simulink model "SAR_Quad_SITL_3D_v3"  (R2025b)
settings: Solver=ode4  StartTime=0.0  StopTime=inf  FixedStep=1/60  RelTol=1e-3
libraries: dspnetwork x5, sim3dlib x1, uavsim3dlib x1
(part 1 of 2)
settings Model: Creator=User  LastModifiedBy=User

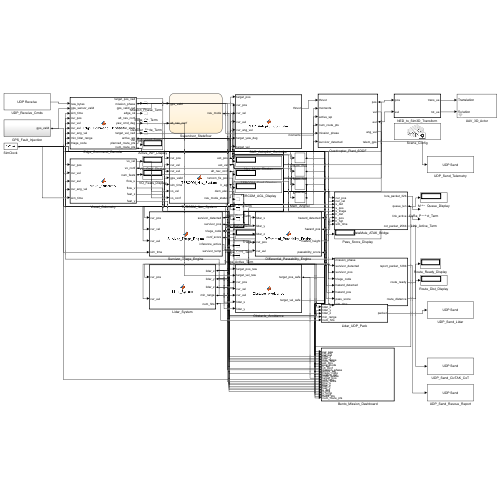
[thumbnail: Simulink's stored preview of the top-level diagram]
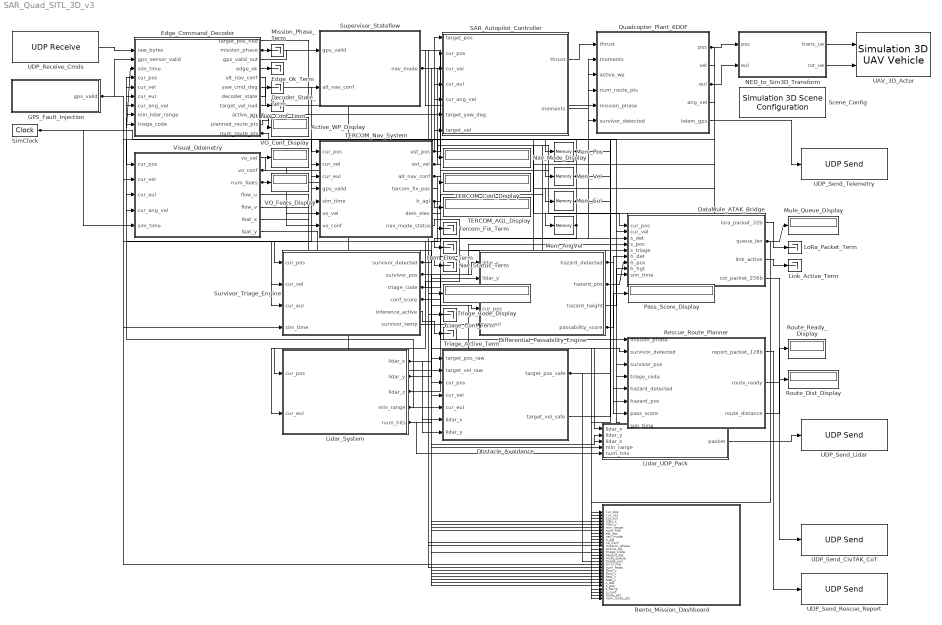
== system SAR_Quad_SITL_3D_v3 ==
  Active_WP_Display : Display
  Alt_Nav_Conf_Term : Terminator
  Bento_Mission_Dashboard : MATLAB Function  TreatAsAtomicUnit=on
  DataMule_ATAK_Bridge : MATLAB Function  TreatAsAtomicUnit=on
  Decoder_State_Term : Terminator
  Dem_Elev_Term : Terminator
  Differential_Passability_Engine : MATLAB Function  TreatAsAtomicUnit=on
  Edge_Command_Decoder : MATLAB Function  TreatAsAtomicUnit=on
  Edge_Ok_Term : Terminator
  GPS_Fault_Injection : Subsystem
  Lidar_System : MATLAB Function  TreatAsAtomicUnit=on
  Lidar_UDP_Pack : MATLAB Function  TreatAsAtomicUnit=on
  Link_Active_Term : Terminator
  LoRa_Packet_Term : Terminator
  Mem_AngVel : Memory  InitialCondition=[0; 0; 0]
  Mem_Eul : Memory  InitialCondition=[0; 0; 0]
  Mem_Pos : Memory  InitialCondition=[0; 0; 0]
  Mem_Vel : Memory  InitialCondition=[0; 0; 0]
  Mission_Phase_Term : Terminator
  Mule_Queue_Display : Display
  NED_to_Sim3D_Transform : MATLAB Function  TreatAsAtomicUnit=on
  Nav_Mode_Display : Display
  Nav_Status_Term : Terminator
  Obstacle_Avoidance : MATLAB Function  TreatAsAtomicUnit=on
  Pass_Score_Display : Display
  Quadcopter_Plant_6DOF : MATLAB Function  TreatAsAtomicUnit=on
  Rescue_Route_Planner : MATLAB Function  TreatAsAtomicUnit=on
  Route_Dist_Display : Display
  Route_Ready_Display : Display
  SAR_Autopilot_Controller : MATLAB Function  TreatAsAtomicUnit=on
  Scene_Config : sim3dlib/Simulation 3D Scene Configuration  Priority=0  ProjectFormat=Default Scenes  SceneDesc=US city block  ProjectName=D:\MLAB\toolbox\shared\sim3d_projects\automotive_project_windows\UE\WindowsNoEditor\VehicleSimulation.exe  ScenePath=/Game/Maps/USCityBlock  EnableOpenDRIVE=off  vehTagList={'Custom';'Scene Origin'}  vehTag=Scene Origin  AttachedCameraRelativeTranslation=[0 0 0]  FreeCameraDefaultInitialTranslation=[-6, 0, 2]  AttachedCameraRelativeRotation=[0 0 0]  FreeCameraDefaultInitialRotation=[0, -15, 0]  ViewpointName=Custom  FreeCameraInitialTranslation=[0, 0, 0]  ViewpointTranslation=[0, 0, 0]  FreeCameraInitialRotation=[0, 0, 0]  ViewpointRotation=[0, 0, 0]  OpVisEn=off  Ts=1/60  EnableWindow=on  EnableRemoteAccess=off  EnableWeather=off  SunAzimuth=90  SunAltitude=40.0  EnableGeospatialSun=off  Latitude=0  Longitude=0  Date=2023-01-01  Time=10:30:00  GeoTimeZone=-5.0  SunDaylightSaving=off  wind=1  clouds=10  EnableVolumetricClouds=off  CloudCoverage=0  CloudAltitude=6  fog=0  rain=0  RaindropsEffect=off  SnowDensity=0  EnableGeospatial=off  TilesetSource=Earth terrain  UseTrueOrigin=off  OriginHeight=200  OriginLatitude=40.744652  OriginLongitude=-73.988864  MapStyle=Aerial  AdditionalAssetIDs=[]  UseAdvancedSunSky=off  SolarTime=11  TimeZone=-5  Day=21  Month=9  Year=2022  UseDaylightSavingTime=on  DSTStartDay=10  DSTStartMonth=3  DSTEndDay=3  DSTEndMonth=11  DSTSwitchHour=2  sensorTag=MainCamera1  sensorId=1  sensorName=MainCamera1  mountLoc=Origin  offsetFlag=off  tmountOffset=[0, 0, 0]  rmountOffset=[0, 0, 0]  HorizontalResolution=1280  VerticalResolution=720  HorizontalFOV=60  mountPoint=[0 0 0]  mountOrientation=[0 0 0]  aMode=4  ID=1  GeoTrigger=Inactive  ViewNameList={'Custom'}  ViewTranslationList={'[0 0 0]'}  ViewRotationList={'[0 0 0]'}
      settings: LibrarySourceBlock=uavsim3dlib/Simulation 3D Scene Configuration
  SimClock : DigitalClock  SampleTime=1/60
  Supervisor_Stateflow : Stateflow chart  TreatAsAtomicUnit=on
  Survivor_Triage_Engine : MATLAB Function  TreatAsAtomicUnit=on
  TERCOM_AGL_Display : Display
  TERCOM_Conf_Display : Display
  TERCOM_Nav_System : MATLAB Function  TreatAsAtomicUnit=on
  Tercom_Fix_Term : Terminator
  Triage_Active_Term : Terminator
  Triage_Code_Display : Display
  Triage_Conf_Term : Terminator
  UAV_3D_Actor : uavsim3dlib/Simulation 3D UAV Vehicle  Priority=-1  Mesh=Quadrotor  MeshPath=/MathWorksUAVContent/UAVs/HexaRotorUAV/HexaRotor.HexaRotor  Color=Black  ActorName=SimulinkVehicle1  UseGlobalFrame=off  InitialTranslation=[0 0 0]  InitialRotation=[0 0 0]  InitialTranslationGlobal=[0 0 0]  InitialGeoOrigin=[0 0 0]  InitialRotationGlobal=[0 0 0]  SampleTime=-1  ActorType=SimulinkVehicle  ID=1  aMode=4  ActorTag=SimulinkVehicle1
  UDP_Receive_Cmds : dspnetwork/UDP Receive  localURL='0.0.0.0'  localPort=5001  remoteURL='0.0.0.0'  remotePort=-1  recvBufferSize=8192  dims=255  signalDatatype=uint8  isComplex=off  isVarSize=on  showBlockingTime=off  blockingTime=0  sampletime=1/60  blockPlatform=[]
  UDP_Send_CivTAK_CoT : dspnetwork/UDP Send  remoteURL='127.0.0.1'  remotePort=4242  localURL='0.0.0.0'  localPortSource=Automatically determine  localPort=2048  sendBufferSize=8192  sampletime=-1  blockPlatform=[]  separateLengthPort=0
  UDP_Send_Lidar : dspnetwork/UDP Send  remoteURL='127.0.0.1'  remotePort=5003  localURL='0.0.0.0'  localPortSource=Automatically determine  localPort=2048  sendBufferSize=8192  sampletime=-1  blockPlatform=[]  separateLengthPort=0
  UDP_Send_Rescue_Report : dspnetwork/UDP Send  remoteURL='127.0.0.1'  remotePort=4243  localURL='0.0.0.0'  localPortSource=Automatically determine  localPort=2048  sendBufferSize=8192  sampletime=-1  blockPlatform=[]  separateLengthPort=0
  UDP_Send_Telemetry : dspnetwork/UDP Send  remoteURL='127.0.0.1'  remotePort=5002  localURL='0.0.0.0'  localPortSource=Automatically determine  localPort=2048  sendBufferSize=8192  sampletime=-1  blockPlatform=[]  separateLengthPort=0
  VO_Conf_Display : Display
  VO_Feats_Display : Display
  Visual_Odometry : MATLAB Function  TreatAsAtomicUnit=on
  wires:
  UDP_Receive_Cmds/1 -> Edge_Command_Decoder/1(raw_bytes)
  GPS_Fault_Injection/1(gps_valid) -> Edge_Command_Decoder/2(gps_sensor_valid), TERCOM_Nav_System/4(gps_valid)
  SimClock/1 -> Edge_Command_Decoder/3(sim_time), Visual_Odometry/5(sim_time), TERCOM_Nav_System/5(sim_time), Survivor_Triage_Engine/4(sim_time), DataMule_ATAK_Bridge/9(sim_time), Rescue_Route_Planner/8(sim_time), Bento_Mission_Dashboard/18(sim_time)
  TERCOM_Nav_System/1(est_pos) -> Edge_Command_Decoder/4(cur_pos), Survivor_Triage_Engine/1(cur_pos), Differential_Passability_Engine/4(cur_pos), DataMule_ATAK_Bridge/1(cur_pos), Obstacle_Avoidance/3(cur_pos), SAR_Autopilot_Controller/2(cur_pos), Bento_Mission_Dashboard/8(est_pos)
  TERCOM_Nav_System/2(est_vel) -> Edge_Command_Decoder/5(cur_vel), Survivor_Triage_Engine/2(cur_vel), DataMule_ATAK_Bridge/2(cur_vel), Obstacle_Avoidance/4(cur_vel), SAR_Autopilot_Controller/3(cur_vel)
  Mem_Eul/1 -> Edge_Command_Decoder/6(cur_eul), Visual_Odometry/3(cur_eul), TERCOM_Nav_System/3(cur_eul), Survivor_Triage_Engine/3(cur_eul), Differential_Passability_Engine/5(cur_eul), Obstacle_Avoidance/5(cur_eul), SAR_Autopilot_Controller/4(cur_eul), Lidar_System/2(cur_eul), Bento_Mission_Dashboard/3(cur_eul)
  Mem_AngVel/1 -> Edge_Command_Decoder/7(cur_ang_vel), Visual_Odometry/4(cur_ang_vel), SAR_Autopilot_Controller/5(cur_ang_vel)
  Lidar_System/4(min_range) -> Edge_Command_Decoder/8(min_lidar_range), Lidar_UDP_Pack/4(min_range), Bento_Mission_Dashboard/6(min_range)
  Survivor_Triage_Engine/3(triage_code) -> Edge_Command_Decoder/9(triage_code), Triage_Code_Display/1, DataMule_ATAK_Bridge/5(s_triage), Rescue_Route_Planner/4(triage_code), Bento_Mission_Dashboard/14(triage_code)
  Edge_Command_Decoder/2(mission_phase) -> Mission_Phase_Term/1, Rescue_Route_Planner/1(mission_phase), Quadcopter_Plant_6DOF/5(mission_phase), Bento_Mission_Dashboard/12(mission_phase)
  Edge_Command_Decoder/3(gps_valid_out) -> Supervisor_Stateflow/1(gps_valid)
  Edge_Command_Decoder/4(edge_ok) -> Edge_Ok_Term/1
  Edge_Command_Decoder/5(alt_nav_conf) -> Alt_Nav_Conf_Term/1
  Edge_Command_Decoder/7(decoder_state) -> Decoder_State_Term/1
  Edge_Command_Decoder/9(active_wp) -> Active_WP_Display/1, Quadcopter_Plant_6DOF/3(active_wp), Bento_Mission_Dashboard/13(active_wp)
  Supervisor_Stateflow/1(nav_mode) -> Nav_Mode_Display/1, Bento_Mission_Dashboard/9(nav_mode)
  TERCOM_Nav_System/3(alt_nav_conf) -> Supervisor_Stateflow/2(alt_nav_conf), TERCOM_Conf_Display/1
  Mem_Pos/1 -> Visual_Odometry/1(cur_pos), TERCOM_Nav_System/1(cur_pos), Lidar_System/1(cur_pos), Bento_Mission_Dashboard/1(cur_pos)
  Mem_Vel/1 -> Visual_Odometry/2(cur_vel), TERCOM_Nav_System/2(cur_vel), Bento_Mission_Dashboard/2(cur_vel)
  Visual_Odometry/2(vo_conf) -> VO_Conf_Display/1, TERCOM_Nav_System/7(vo_conf), Bento_Mission_Dashboard/11(vo_conf)
  Visual_Odometry/3(num_feats) -> VO_Feats_Display/1, Bento_Mission_Dashboard/19(num_feats)
  Visual_Odometry/1(vo_vel) -> TERCOM_Nav_System/6(vo_vel)
  TERCOM_Nav_System/4(tercom_fix_pos) -> Tercom_Fix_Term/1
  TERCOM_Nav_System/5(h_agl) -> TERCOM_AGL_Display/1, Bento_Mission_Dashboard/10(h_agl)
  TERCOM_Nav_System/6(dem_elev) -> Dem_Elev_Term/1
  TERCOM_Nav_System/7(nav_mode_status) -> Nav_Status_Term/1
  Survivor_Triage_Engine/4(conf_score) -> Triage_Conf_Term/1, Bento_Mission_Dashboard/27(s_conf)
  Survivor_Triage_Engine/5(inference_active) -> Triage_Active_Term/1
  Lidar_System/1(lidar_x) -> Differential_Passability_Engine/1(lidar_x), Obstacle_Avoidance/6(lidar_x), Lidar_UDP_Pack/1(lidar_x), Bento_Mission_Dashboard/4(lidar_x)
  Lidar_System/2(lidar_y) -> Differential_Passability_Engine/2(lidar_y), Obstacle_Avoidance/7(lidar_y), Lidar_UDP_Pack/2(lidar_y), Bento_Mission_Dashboard/5(lidar_y)
  Lidar_System/3(lidar_z) -> Differential_Passability_Engine/3(lidar_z), Lidar_UDP_Pack/3(lidar_z)
  Differential_Passability_Engine/4(passability_score) -> Pass_Score_Display/1, Rescue_Route_Planner/7(pass_score)
  Survivor_Triage_Engine/1(survivor_detected) -> DataMule_ATAK_Bridge/3(s_det), Rescue_Route_Planner/2(survivor_detected), Quadcopter_Plant_6DOF/6(survivor_detected), Bento_Mission_Dashboard/24(s_det)
  Survivor_Triage_Engine/2(survivor_pos) -> DataMule_ATAK_Bridge/4(s_pos), Rescue_Route_Planner/3(survivor_pos), Bento_Mission_Dashboard/25(s_pos)
  Differential_Passability_Engine/1(hazard_detected) -> DataMule_ATAK_Bridge/6(h_det), Rescue_Route_Planner/5(hazard_detected), Bento_Mission_Dashboard/15(hazard_det)
  Differential_Passability_Engine/2(hazard_pos) -> DataMule_ATAK_Bridge/7(h_pos), Rescue_Route_Planner/6(hazard_pos)
  Differential_Passability_Engine/3(hazard_height) -> DataMule_ATAK_Bridge/8(h_hgt)
  DataMule_ATAK_Bridge/1(lora_packet_32b) -> LoRa_Packet_Term/1
  DataMule_ATAK_Bridge/2(queue_len) -> Mule_Queue_Display/1, Bento_Mission_Dashboard/16(mule_queue)
  DataMule_ATAK_Bridge/3(link_active) -> Link_Active_Term/1
  DataMule_ATAK_Bridge/4(cot_packet_256b) -> UDP_Send_CivTAK_CoT/1
  Rescue_Route_Planner/1(report_packet_128b) -> UDP_Send_Rescue_Report/1
  Rescue_Route_Planner/2(route_ready) -> Route_Ready_Display/1
  Rescue_Route_Planner/3(route_distance) -> Route_Dist_Display/1
  Edge_Command_Decoder/1(target_pos_ned) -> Obstacle_Avoidance/1(target_pos_raw)
  Edge_Command_Decoder/8(target_vel_ned) -> Obstacle_Avoidance/2(target_vel_raw)
  Obstacle_Avoidance/1(target_pos_safe) -> SAR_Autopilot_Controller/1(target_pos), Bento_Mission_Dashboard/17(target_pos)
  Edge_Command_Decoder/6(yaw_cmd_deg) -> SAR_Autopilot_Controller/6(target_yaw_deg)
  Obstacle_Avoidance/2(target_vel_safe) -> SAR_Autopilot_Controller/7(target_vel)
  SAR_Autopilot_Controller/1(thrust) -> Quadcopter_Plant_6DOF/1(thrust)
  SAR_Autopilot_Controller/2(moments) -> Quadcopter_Plant_6DOF/2(moments)
  Edge_Command_Decoder/11(num_route_pts) -> Quadcopter_Plant_6DOF/4(num_route_pts), Bento_Mission_Dashboard/29(num_route_pts)
  Quadcopter_Plant_6DOF/1(pos) -> Mem_Pos/1, NED_to_Sim3D_Transform/1(pos)
  Quadcopter_Plant_6DOF/2(vel) -> Mem_Vel/1
  Quadcopter_Plant_6DOF/3(eul) -> Mem_Eul/1, NED_to_Sim3D_Transform/2(eul)
  Quadcopter_Plant_6DOF/4(ang_vel) -> Mem_AngVel/1
  Lidar_System/5(num_hits) -> Lidar_UDP_Pack/5(num_hits), Bento_Mission_Dashboard/7(num_hits)
  Lidar_UDP_Pack/1(packet) -> UDP_Send_Lidar/1
  NED_to_Sim3D_Transform/1(trans_ue) -> UAV_3D_Actor/1
  NED_to_Sim3D_Transform/2(rot_ue) -> UAV_3D_Actor/2
  Quadcopter_Plant_6DOF/5(telem_gps) -> UDP_Send_Telemetry/1
  Visual_Odometry/4(flow_u) -> Bento_Mission_Dashboard/20(flow_u)
  Visual_Odometry/5(flow_v) -> Bento_Mission_Dashboard/21(flow_v)
  Visual_Odometry/6(feat_x) -> Bento_Mission_Dashboard/22(feat_x)
  Visual_Odometry/7(feat_y) -> Bento_Mission_Dashboard/23(feat_y)
  Survivor_Triage_Engine/6(survivor_temp) -> Bento_Mission_Dashboard/26(s_temp)
  Edge_Command_Decoder/10(planned_route_pts) -> Bento_Mission_Dashboard/28(route_pts)

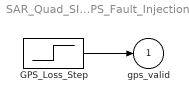
== system SAR_Quad_SITL_3D_v3/GPS_Fault_Injection ==
  GPS_Loss_Step : Step  Time=160  Before=1  After=0  SampleTime=1/60
  gps_valid : Outport
  wires:
  ? -> ?
  GPS_Loss_Step/1 -> gps_valid/1

== matlab function SAR_Quad_SITL_3D_v3/Survivor_Triage_Engine ==
  data: cur_pos input; survivor_detected output size=1; cur_vel input; cur_eul input; sim_time input; survivor_pos output size=3; triage_code output size=1; conf_score output size=1; inference_active output size=1; survivor_temp output size=1
function [survivor_detected, survivor_pos, triage_code, conf_score, inference_active, survivor_temp] = Survivor_Triage_Engine(cur_pos, cur_vel, cur_eul, sim_time)
survivor_detected = 0.0;
survivor_pos = [0.0; 0.0; 0.0];
triage_code = 0.0; conf_score = 0.0; inference_active = 0.0;
AMBIENT_TEMP = 22.0;
survivor_temp = AMBIENT_TEMP;
persistent survivors
if isempty(survivors)
    survivors = [
        145.0,  50.0, 0.0, 38.2, 1.0;   % Park Sector Target Actor (RED IMMEDIATE)
         22.0,   5.5, 0.0, 37.4, 1.0;   % Sector 1: Immediate Critical (RED)
        120.0, -35.0, 0.0, 36.8, 2.0;   % Sector 2: Delayed Triage (YELLOW)
         50.0,  18.0, 0.0, 36.9, 3.0    % Sector 3: Minor Injury (GREEN)
    ];
end
h_agl = max(1.0, -cur_pos(3));
r_footprint = max(4.5, h_agl * tan(35.0 * pi / 180));
v_ground = norm(cur_vel(1:2));

for i = 1:size(survivors, 1)
    d_xy = norm(survivors(i, 1:2) - cur_pos(1:2)');
    if d_xy <= r_footprint && h_agl >= 1.5
        inference_active = 1.0;
        survivor_detected = 1.0;
        survivor_pos = survivors(i, 1:3)';
        triage_code = survivors(i, 5);
        survivor_temp = survivors(i, 4);
        conf_score = max(0.60, 0.98 - 0.03 * (d_xy / r_footprint) - 0.01 * v_ground);
        break;
    end
end

== matlab function SAR_Quad_SITL_3D_v3/Differential_Passability_Engine ==
  data: lidar_x input; hazard_detected output size=1; lidar_y input; lidar_z input; cur_pos input; cur_eul input; hazard_pos output size=3; hazard_height output size=1; passability_score output size=1
function [hazard_detected, hazard_pos, hazard_height, passability_score] = Differential_Passability_Engine(lidar_x, lidar_y, lidar_z, cur_pos, cur_eul)
hazard_detected = 0.0;
hazard_pos = [0.0; 0.0; 0.0];
hazard_height = 0.0;
passability_score = 1.0;
yaw = cur_eul(3); c = cos(yaw); s = sin(yaw);
wx = cur_pos(1) + c .* lidar_x - s .* lidar_y;
wy = cur_pos(2) + s .* lidar_x + c .* lidar_y;
wz = -cur_pos(3) + lidar_z;
N = numel(lidar_x);
max_delta = 0.0; best_hx = 0.0; best_hy = 0.0;
for i = 1:min(N, 72)
    is_road = (abs(wy(i)) <= 7.5) || (abs(wx(i) - 120.0) <= 7.5) || (abs(wx(i) - 50.0) <= 4.0) || (abs(wx(i) + 20.0) <= 7.5);
    if is_road && wz(i) > 0.35 && wz(i) < 4.0
        if wz(i) > max_delta
            max_delta = wz(i); best_hx = wx(i); best_hy = wy(i);
        end
    end
end
if max_delta > 0.40
    hazard_detected = 1.0;
    hazard_pos = [best_hx; best_hy; max_delta];
    hazard_height = max_delta;
    passability_score = max(0.0, 1.0 - (max_delta / 3.0));
end

== matlab function SAR_Quad_SITL_3D_v3/DataMule_ATAK_Bridge ==
  data: cur_pos input; lora_packet_32b output size=32; cur_vel input; s_det input; s_pos input; s_triage input; h_det input; h_pos input; h_hgt input; sim_time input; queue_len output size=1; link_active output size=1; cot_packet_256b output size=256
function [lora_packet_32b, queue_len, link_active, cot_packet_256b] = DataMule_ATAK_Bridge(cur_pos, cur_vel, s_det, s_pos, s_triage, h_det, h_pos, h_hgt, sim_time)
lora_packet_32b = zeros(32, 1, 'uint8');
cot_packet_256b = zeros(256, 1, 'uint8');
link_active = 0.0;
persistent queue_count cot_count
if isempty(queue_count)
    queue_count = 0.0; cot_count = 0.0;
end
if norm(cur_pos(1:2)) < 40.0; link_active = 1.0; end
if s_det > 0.5 || h_det > 0.5; queue_count = min(64.0, queue_count + 0.05); end
if link_active > 0.5 && queue_count > 0.1
    queue_count = max(0.0, queue_count - 0.25);
    cot_count   = cot_count + 1.0;
end

lora_packet_32b(1) = uint8(170);
lora_packet_32b(2) = uint8(s_triage);
lora_packet_32b(3) = uint8(round(min(30.0, norm(cur_vel(1:2))) * 10));
lora_packet_32b(4) = uint8(round(min(50.0, -cur_pos(3))));
lora_packet_32b(5) = uint8(round(h_hgt * 10));
lora_packet_32b(6) = uint8(mod(round(sim_time), 255));
lora_packet_32b(7) = uint8(round(max(0.0, min(100.0, 98.0 - sim_time * 0.05))));

cot_msg = sprintf('<event version="2.0" uid="SAR-UAV-01" type="a-f-G-U-C" how="m-g" time="%.0f" start="%.0f" stale="%.0f"><point lat="26.9948" lon="88.2854" hae="%.1f" ce="1.5" le="1.0"/><detail><triage code="%.0f"/><contact callsign="RESCUE-BRAIN-01"/></detail></event>', sim_time, sim_time, sim_time + 30, -cur_pos(3), s_triage);
bytes = uint8(cot_msg);
n = min(numel(bytes), 256);
cot_packet_256b(1:n) = bytes(1:n);
queue_len = queue_count;

== matlab function SAR_Quad_SITL_3D_v3/Rescue_Route_Planner ==
  data: mission_phase input; report_packet_128b output size=128; survivor_detected input; survivor_pos input; triage_code input; hazard_detected input; hazard_pos input; pass_score input; sim_time input; route_ready output size=1; route_distance output size=1
function [report_packet_128b, route_ready, route_distance] = Rescue_Route_Planner(mission_phase, survivor_detected, survivor_pos, triage_code, hazard_detected, hazard_pos, pass_score, sim_time)
report_packet_128b = zeros(128, 1, 'uint8');
route_ready = 0.0; route_distance = 0.0;
MAX_WP = 6; route_pts = zeros(MAX_WP, 2); num_pts = 0.0;
if mission_phase >= 1.0 || survivor_detected > 0.5
    route_ready = 1.0;
    dest_north = 145.0; dest_east = 50.0;
    if survivor_detected > 0.5
        dest_north = survivor_pos(1); dest_east = survivor_pos(2);
    end
    p_base = [0.0, 0.0]; p_target = [dest_north, dest_east];
    detour_needed = false;
    if hazard_detected > 0.5
        if norm(hazard_pos(1:2) - [60.0; 0.0]) < 10.0; detour_needed = true; end
    end
    if detour_needed
        route_pts(1, :) = p_base; route_pts(2, :) = [20.0, -4.5]; route_pts(3, :) = [120.0, -4.5]; route_pts(4, :) = p_target;
        num_pts = 4.0; mode_flag = 2.0;
    else
        route_pts(1, :) = p_base; route_pts(2, :) = [dest_north, 0.0]; route_pts(3, :) = p_target;
        num_pts = 3.0; mode_flag = 1.0;
    end
    total_d = 0.0;
    for i = 1:(int32(num_pts) - 1)
        total_d = total_d + norm(route_pts(i+1, :) - route_pts(i, :));
    end
    route_distance = total_d;
    msg = sprintf('RPT:INGRESS|TGT:%.0f,%.0f|TRG:%.0f|DIST:%.1fm|DETOUR:%.0f|WP_CNT:%.0f|TIME:%.0f', dest_north, dest_east, triage_code, route_distance, mode_flag, num_pts, sim_time);
    b_str = uint8(msg); n_len = min(numel(b_str), 128);
    report_packet_128b(1:n_len) = b_str(1:n_len);
end

== matlab function SAR_Quad_SITL_3D_v3/SAR_Autopilot_Controller ==
  data: target_pos input; thrust output size=1; cur_pos input; cur_vel input; cur_eul input; cur_ang_vel input; target_yaw_deg input; target_vel input; moments output size=3
function [thrust, moments] = SAR_Autopilot_Controller(target_pos, cur_pos, cur_vel, cur_eul, cur_ang_vel, target_yaw_deg, target_vel)
thrust = 0.0; moments = [0.0; 0.0; 0.0];
persistent int_vel_err int_att_err int_z_err
persistent pitch_cmd_filt roll_cmd_filt
if isempty(int_vel_err)
    int_vel_err = [0.0; 0.0]; int_att_err = [0.0; 0.0; 0.0]; int_z_err = 0.0;
    pitch_cmd_filt = 0.0; roll_cmd_filt = 0.0;
end

if cur_pos(3) >= -0.05 && target_pos(3) >= -0.05
    thrust = 0.0;
    moments = [0.0; 0.0; 0.0];
    int_vel_err = [0.0; 0.0]; int_att_err = [0.0; 0.0; 0.0]; int_z_err = 0.0;
    pitch_cmd_filt = 0.0; roll_cmd_filt = 0.0;
    return;
end

dt = 1/60; m = 1.8; g = 9.81;

% REALISTIC TACTICAL TILT LIMIT (20 DEGREES)
kp_p = 1.90; kp_v = 3.40; ki_v = 0.14;
e_pos_xy = target_pos(1:2) - cur_pos(1:2);
e_vel_xy = target_vel(1:2) - cur_vel(1:2);
int_vel_err = max(min(int_vel_err + (e_vel_xy * dt), 0.8), -0.8);

acc_world = kp_p * e_pos_xy + kp_v * e_vel_xy + ki_v * int_vel_err;
yaw_now = cur_eul(3);
acc_body_x =  acc_world(1) * cos(yaw_now) + acc_world(2) * sin(yaw_now);
acc_body_y = -acc_world(1) * sin(yaw_now) + acc_world(2) * cos(yaw_now);

MAX_TILT = 20.0 * pi / 180.0; % Hard mechanical bank ceiling
pitch_cmd_raw = max(min(-acc_body_x / g, MAX_TILT), -MAX_TILT);
roll_cmd_raw  = max(min( acc_body_y / g, MAX_TILT), -MAX_TILT);

% TILT FILTER (Smooth 10 Hz roll/pitch response)
alpha_tilt = 0.14;
pitch_cmd_filt = (1.0 - alpha_tilt) * pitch_cmd_filt + alpha_tilt * pitch_cmd_raw;
roll_cmd_filt  = (1.0 - alpha_tilt) * roll_cmd_filt  + alpha_tilt * roll_cmd_raw;

kp_z = 7.50; ki_z = 0.60; kd_z = 3.80;
e_pos_z = target_pos(3) - cur_pos(3);
e_vel_z = target_vel(3) - cur_vel(3);
int_z_err = max(min(int_z_err + (e_pos_z * dt), 1.2), -1.2);
az_pid = kp_z * e_pos_z + kd_z * e_vel_z + ki_z * int_z_err;
az_cmd = max(-10.0, min(0.50 * g, az_pid));

cos_tilt = cos(cur_eul(1)) * cos(cur_eul(2));
cos_tilt_safe = max(0.70, cos_tilt);
thrust_raw = m * (g - az_cmd) / cos_tilt_safe;
thrust = max(0.40 * m * g, min(thrust_raw, 2.80 * m * g));

% DAMPED, JITTER-FREE INNER ATTITUDE LOOP
kp_att = [5.50; 5.50; 2.60];
ki_att = [0.08; 0.08; 0.03];
kd_att = [0.40; 0.40; 0.30];

yaw_target_rad = target_yaw_deg * pi / 180.0;
yaw_err = atan2(sin(yaw_target_rad - cur_eul(3)), cos(yaw_target_rad - cur_eul(3)));
att_err = [roll_cmd_filt - cur_eul(1); pitch_cmd_filt - cur_eul(2); yaw_err];
int_att_err = max(min(int_att_err + (att_err * dt), 0.15), -0.15);
moments = kp_att .* att_err + ki_att .* int_att_err - kd_att .* cur_ang_vel;
moments = max(min(moments, 2.2), -2.2);

== matlab function SAR_Quad_SITL_3D_v3/Quadcopter_Plant_6DOF ==
  data: thrust input; pos output size=3; moments input; active_wp input; num_route_pts input; mission_phase input; survivor_detected input; vel output size=3; eul output size=3; ang_vel output size=3; telem_gps output size=20
function [pos, vel, eul, ang_vel, telem_gps] = Quadcopter_Plant_6DOF(thrust, moments, active_wp, num_route_pts, mission_phase, survivor_detected)
pos = zeros(3, 1); vel = zeros(3, 1); eul = zeros(3, 1); ang_vel = zeros(3, 1); telem_gps = zeros(20, 1);
persistent p v e w buildings
if isempty(p)
    p = [0; 0; 0]; v = [0; 0; 0]; e = [0; 0; 0]; w = [0; 0; 0];
    buildings = [
        -12.5,  46.0,   8.0,  80.0, -35.0, 0.0;   % Northwest Block 1
         54.0, 111.0,   8.0,  80.0, -35.0, 0.0;   % Northwest Block 2 (Red brick building)
        -12.5,  46.0, -80.0,  -8.0, -35.0, 0.0;   % Southwest Block 1
         54.0, 111.0, -80.0,  -8.0, -35.0, 0.0;   % Southwest Block 2
        195.0, 255.0,   8.0,  80.0, -35.0, 0.0;   % Far East Block
        129.0, 200.0, -80.0,  -8.0, -35.0, 0.0;   % Southeast Block
        -80.0, -29.0,   8.0,  80.0, -35.0, 0.0;   % West-North Block
        -80.0, -29.0, -80.0,  -8.0, -35.0, 0.0    % West-South Block
    ];
end
dt = 1/60; m = 1.8; g = 9.81;
I = diag([0.02, 0.02, 0.04]);
phi = e(1); theta = e(2); psi = e(3);
R = [cos(theta)*cos(psi), sin(phi)*sin(theta)*cos(psi)-cos(phi)*sin(psi), cos(phi)*sin(theta)*cos(psi)+sin(phi)*sin(psi);
     cos(theta)*sin(psi), sin(phi)*sin(theta)*sin(psi)+cos(phi)*cos(psi), cos(phi)*sin(theta)*sin(psi)-sin(phi)*cos(psi);
    -sin(theta),          sin(phi)*cos(theta),                            cos(phi)*cos(theta)];
f_body = [0; 0; -thrust];
drag_force = -0.05 * norm(v(1:2)) * [v(1); v(2); 0];
acc = (R * f_body + [0; 0; m*g] + drag_force) / m;
v = v + acc * dt; p = p + v * dt;

if p(3) >= -0.05
    p(3) = 0.0;
    if v(3) > 0.0; v(3) = 0.0; end
    v(1:2) = v(1:2) * 0.40;
    if abs(v(3)) < 0.05 && thrust < m*g * 0.95
        e(1) = 0.0; e(2) = 0.0; w(1:3) = [0;0;0];
    end
end

ROBOT_R = 0.45;
for b = 1:size(buildings, 1)
    b_xmin = buildings(b, 1) - ROBOT_R; b_xmax = buildings(b, 2) + ROBOT_R;
    b_ymin = buildings(b, 3) - ROBOT_R; b_ymax = buildings(b, 4) + ROBOT_R;
    b_zmin = buildings(b, 5);           b_zmax = buildings(b, 6);
    if p(1) >= b_xmin && p(1) <= b_xmax && p(2) >= b_ymin && p(2) <= b_ymax && p(3) >= b_zmin && p(3) <= b_zmax
        dx_min = abs(p(1) - b_xmin); dx_max = abs(p(1) - b_xmax);
        dy_min = abs(p(2) - b_ymin); dy_max = abs(p(2) - b_ymax);
        [~, face_idx] = min([dx_min, dx_max, dy_min, dy_max]);
        if face_idx == 1;     p(1) = b_xmin; v(1) = min(0.0, v(1));
        elseif face_idx == 2; p(1) = b_xmax; v(1) = max(0.0, v(1));
        elseif face_idx == 3; p(2) = b_ymin; v(2) = min(0.0, v(2));
        else;                 p(2) = b_ymax; v(2) = max(0.0, v(2));
        end
        v(1:2) = v(1:2) * 0.3;
    end
end

ang_acc = I \ (moments - cross(w, I * w));
w = max(min(w + ang_acc * dt, 4.0), -4.0);
T = [1, sin(e(1))*tan(e(2)), cos(e(1))*tan(e(2)); 0, cos(e(1)), -sin(e(1)); 0, sin(e(1))/cos(e(2)), cos(e(1))/cos(e(2))];
e = e + (T * w) * dt;

MAX_SAFE_ROLL = 24.0 * pi / 180.0;
MAX_SAFE_PITCH = 24.0 * pi / 180.0;
if abs(e(1)) > MAX_SAFE_ROLL; e(1) = sign(e(1)) * MAX_SAFE_ROLL; w(1) = 0.0; end
if abs(e(2)) > MAX_SAFE_PITCH; e(2) = sign(e(2)) * MAX_SAFE_PITCH; w(2) = 0.0; end
e(3) = atan2(sin(e(3)), cos(e(3)));

pos = p; vel = v; eul = e; ang_vel = w;
ref_lat = 26.99484; ref_lon = 88.28542;
lat = ref_lat + (p(1) / 111320.0);
lon = ref_lon + (p(2) / (111320.0 * cos(ref_lat * pi / 180)));

% 20-DOUBLE CLOSED-LOOP TELEMETRY PACKET
telem_gps(1)  = lat;
telem_gps(2)  = lon;
telem_gps(3)  = -p(3);
telem_gps(4)  = v(1);
telem_gps(5)  = v(2);
telem_gps(6)  = v(3);
telem_gps(7)  = e(1);
telem_gps(8)  = e(2);
telem_gps(9)  = e(3);
telem_gps(10) = w(1);
telem_gps(11) = w(2);
telem_gps(12) = w(3);
telem_gps(13) = p(1);
telem_gps(14) = p(2);
telem_gps(15) = p(3);
telem_gps(16) = thrust;
telem_gps(17) = active_wp;          % Real-time pattern index
telem_gps(18) = num_route_pts;      % Total pattern legs
telem_gps(19) = mission_phase;      % Active flight mode
telem_gps(20) = survivor_detected;  % YOLO target lock status

== matlab function SAR_Quad_SITL_3D_v3/Lidar_System ==
  data: cur_pos input; lidar_x output size=108; cur_eul input; lidar_y output size=108; lidar_z output size=108; min_range output size=1; num_hits output size=1
function [lidar_x, lidar_y, lidar_z, min_range, num_hits] = Lidar_System(cur_pos, cur_eul)
N_AZ = 36; ELEVS = [-15, 0, 15] * pi / 180; N_EL = numel(ELEVS); N = N_AZ * N_EL;
MAX_RANGE = 30.0;
lidar_x = zeros(N, 1); lidar_y = zeros(N, 1); lidar_z = zeros(N, 1);
min_range = MAX_RANGE; num_hits = 0.0;
persistent buildings
if isempty(buildings)
    buildings = [
        -12.5,  46.0,   8.0,  80.0, -35.0, 0.0;   % Northwest Block 1
         54.0, 111.0,   8.0,  80.0, -35.0, 0.0;   % Northwest Block 2 (Red brick building)
        -12.5,  46.0, -80.0,  -8.0, -35.0, 0.0;   % Southwest Block 1
         54.0, 111.0, -80.0,  -8.0, -35.0, 0.0;   % Southwest Block 2
        195.0, 255.0,   8.0,  80.0, -35.0, 0.0;   % Far East Block
        129.0, 200.0, -80.0,  -8.0, -35.0, 0.0;   % Southeast Block
        -80.0, -29.0,   8.0,  80.0, -35.0, 0.0;   % West-North Block
        -80.0, -29.0, -80.0,  -8.0, -35.0, 0.0    % West-South Block
    ];
end

az_body = (-pi + (0:N_AZ-1) * (2*pi/N_AZ))';
az_rep = repmat(az_body, N_EL, 1); el_rep = repelem(ELEVS(:), N_AZ);
dx_b = cos(az_rep) .* cos(el_rep); dy_b = sin(az_rep) .* cos(el_rep); dz_b = -sin(el_rep);

yaw = cur_eul(3); c = cos(yaw); s = sin(yaw);
dx_w = c * dx_b - s * dy_b; dy_w = s * dx_b + c * dy_b; dz_w = dz_b;

ox = cur_pos(1); oy = cur_pos(2); oz = cur_pos(3);
best_t = MAX_RANGE * ones(N, 1); hit_flags = false(N, 1);

for r = 1:N
    rx = dx_w(r); ry = dy_w(r); rz = dz_w(r);
    for b = 1:size(buildings, 1)
        bx1 = buildings(b, 1); bx2 = buildings(b, 2);
        by1 = buildings(b, 3); by2 = buildings(b, 4);
        bz1 = buildings(b, 5); bz2 = buildings(b, 6);
        if abs(rx) > 1e-5
            tx1 = (bx1 - ox) / rx; tx2 = (bx2 - ox) / rx;
            tmin_x = min(tx1, tx2); tmax_x = max(tx1, tx2);
        else
            if ox >= bx1 && ox <= bx2; tmin_x = -1e6; tmax_x = 1e6;
            else;                      tmin_x = 1e6;  tmax_x = -1e6; end
        end
        if abs(ry) > 1e-5
            ty1 = (by1 - oy) / ry; ty2 = (by2 - oy) / ry;
            tmin_y = min(ty1, ty2); tmax_y = max(ty1, ty2);
        else
            if oy >= by1 && oy <= by2; tmin_y = -1e6; tmax_y = 1e6;
            else;                      tmin_y = 1e6;  tmax_y = -1e6; end
        end
        if abs(rz) > 1e-5
            tz1 = (bz1 - oz) / rz; tz2 = (bz2 - oz) / rz;
            tmin_z = min(tz1, tz2); tmax_z = max(tz1, tz2);
        else
            if oz >= bz1 && oz <= bz2; tmin_z = -1e6; tmax_z = 1e6;
            else;                      tmin_z = 1e6;  tmax_z = -1e6; end
        end
        t_enter = max(max(tmin_x, tmin_y), tmin_z);
        t_exit  = min(min(tmax_x, tmax_y), tmax_z);
        if t_exit >= max(0.0, t_enter) && t_enter < best_t(r)
            best_t(r) = t_enter;
            hit_flags(r) = true;
        end
    end
end

lidar_x = best_t .* dx_b;
lidar_y = best_t .* dy_b;
lidar_z = best_t .* dz_b;
num_hits = double(sum(hit_flags));
if any(hit_flags); min_range = min(best_t(hit_flags)); else; min_range = MAX_RANGE; end

== matlab function SAR_Quad_SITL_3D_v3/Obstacle_Avoidance ==
  data: target_pos_raw input; target_pos_safe output size=3; target_vel_raw input; cur_pos input; cur_vel input; cur_eul input; lidar_x input; lidar_y input; target_vel_safe output size=3
function [target_pos_safe, target_vel_safe] = Obstacle_Avoidance(target_pos_raw, target_vel_raw, cur_pos, cur_vel, cur_eul, lidar_x, lidar_y)
target_pos_safe = [target_pos_raw(1); target_pos_raw(2); target_pos_raw(3)];
target_vel_safe = [target_vel_raw(1); target_vel_raw(2); target_vel_raw(3)];

SAFETY_RANGE = 4.8;
CRIT_RANGE   = 1.6;
dt = 1/60;

persistent last_pos stuck_timer unstuck_mode unstuck_timer unstuck_dir
if isempty(stuck_timer)
    last_pos = cur_pos(1:2);
    stuck_timer = 0.0;
    unstuck_mode = 0.0;
    unstuck_timer = 0.0;
    unstuck_dir = [0.0; 0.0];
end

v_est = norm(cur_pos(1:2) - last_pos) / dt;
last_pos = cur_pos(1:2);

to_goal = target_pos_raw(1:2) - cur_pos(1:2);
dist_goal = norm(to_goal);
if dist_goal > 0.01; u_goal = to_goal / dist_goal; else; u_goal = [0.0; 0.0]; end

horiz_dist = sqrt(lidar_x.^2 + lidar_y.^2);
valid = (horiz_dist > 0.3) & (horiz_dist < SAFETY_RANGE);
min_dist = SAFETY_RANGE;
closest_idx = 0;
if any(valid)
    valid_ranges = horiz_dist;
    valid_ranges(~valid) = 1e6;
    [min_dist, closest_idx] = min(valid_ranges);
end

if min_dist < 1.8 && v_est < 0.25 && dist_goal > 0.8
    stuck_timer = stuck_timer + dt;
else
    stuck_timer = max(0.0, stuck_timer - 0.5 * dt);
end

if stuck_timer > 0.40 && unstuck_mode < 0.5
    unstuck_mode = 1.0;
    unstuck_timer = 1.5;
    yaw = cur_eul(3); c = cos(yaw); s = sin(yaw);
    if closest_idx > 0
        wx = c * lidar_x(closest_idx) - s * lidar_y(closest_idx);
        wy = s * lidar_x(closest_idx) + c * lidar_y(closest_idx);
        u_obs = [wx; wy] / max(norm([wx; wy]), 0.1);
    else
        u_obs = [cos(yaw); sin(yaw)];
    end
    u_tang = [-u_obs(2); u_obs(1)];
    if dot(u_tang, u_goal) < 0.0; u_tang = -u_tang; end
    unstuck_dir = -u_obs * 0.80 + u_tang * 0.60;
    unstuck_dir = unstuck_dir / max(norm(unstuck_dir), 0.01);
end

if unstuck_mode > 0.5
    unstuck_timer = unstuck_timer - dt;
    if unstuck_timer <= 0.0 || min_dist > 3.5
        unstuck_mode = 0.0;
        stuck_timer = 0.0;
    else
        target_pos_safe(1) = cur_pos(1) + unstuck_dir(1) * 2.5;
        target_pos_safe(2) = cur_pos(2) + unstuck_dir(2) * 2.5;
        target_pos_safe(3) = target_pos_raw(3);
        target_vel_safe(1) = unstuck_dir(1) * 2.8;
        target_vel_safe(2) = unstuck_dir(2) * 2.8;
        target_vel_safe(3) = target_vel_raw(3);
        return;
    end
end

if closest_idx > 0 && min_dist < SAFETY_RANGE
    yaw = cur_eul(3); c = cos(yaw); s = sin(yaw);
    wx = c * lidar_x(closest_idx) - s * lidar_y(closest_idx);
    wy = s * lidar_x(closest_idx) + c * lidar_y(closest_idx);
    u_obs = [wx; wy] / max(min_dist, 0.1);
    eta = max(0.0, min(1.0, (SAFETY_RANGE - min_dist) / (SAFETY_RANGE - CRIT_RANGE)));
    
    u_tang = [-u_obs(2); u_obs(1)];
    if dot(u_tang, u_goal) < 0.0; u_tang = -u_tang; end
    
    proj_into_obs = dot(u_goal, u_obs);
    if proj_into_obs > 0.0
        u_goal_safe = u_goal - proj_into_obs * u_obs;
        norm_g = norm(u_goal_safe);
        if norm_g > 0.05; u_goal_safe = u_goal_safe / norm_g; else; u_goal_safe = u_tang; end
    else
        u_goal_safe = u_goal;
    end
    
    v_steer = (1.0 - eta) * u_goal_safe + eta * (-u_obs * 0.55 + u_tang * 1.05);
    v_steer = v_steer / max(norm(v_steer), 0.01);
    
    lookahead = min(max(min_dist * 0.85, 2.0), max(dist_goal, 0.8));
    target_pos_safe(1) = cur_pos(1) + v_steer(1) * lookahead;
    target_pos_safe(2) = cur_pos(2) + v_steer(2) * lookahead;
    target_pos_safe(3) = target_pos_raw(3);
    
    v_mag = max(2.2, norm(target_vel_raw(1:2)) * (1.0 - 0.35 * eta));
    target_vel_safe(1) = v_steer(1) * v_mag;
    target_vel_safe(2) = v_steer(2) * v_mag;
    target_vel_safe(3) = target_vel_raw(3);
else
    if dist_goal > 4.5
        target_pos_safe(1) = cur_pos(1) + u_goal(1) * 4.2;
        target_pos_safe(2) = cur_pos(2) + u_goal(2) * 4.2;
    else
        target_pos_safe(1) = target_pos_raw(1);
        target_pos_safe(2) = target_pos_raw(2);
    end
    target_pos_safe(3) = target_pos_raw(3);
    target_vel_safe = target_vel_raw;
end

== matlab function SAR_Quad_SITL_3D_v3/Lidar_UDP_Pack ==
  data: lidar_x input; packet output; lidar_y input; lidar_z input; min_range input; num_hits input
function packet = Lidar_UDP_Pack(lidar_x, lidar_y, lidar_z, min_range, num_hits)
packet = [double(numel(lidar_x)); lidar_x(:); lidar_y(:); lidar_z(:); double(min_range); double(num_hits)];

== matlab function SAR_Quad_SITL_3D_v3/NED_to_Sim3D_Transform ==
  data: pos input; trans_ue output size=3; eul input; rot_ue output size=3
function [trans_ue, rot_ue] = NED_to_Sim3D_Transform(pos, eul)
trans_ue = zeros(3, 1);
rot_ue   = zeros(3, 1);
trans_ue(1) = pos(1);
trans_ue(2) = -pos(2);
trans_ue(3) = -pos(3);
rot_ue(1) = -eul(3);
rot_ue(2) = -eul(2);
rot_ue(3) =  eul(1);

== matlab function SAR_Quad_SITL_3D_v3/Bento_Mission_Dashboard ==
  data: cur_pos input; cur_vel input; cur_eul input; lidar_x input; lidar_y input; min_range input; num_hits input; est_pos input; nav_mode input; h_agl input; vo_conf input; mission_phase input; active_wp input; triage_code input; hazard_det input; mule_queue input; target_pos input; sim_time input; num_feats input; flow_u input; flow_v input; feat_x input; feat_y input; s_det input; s_pos input; s_temp input; s_conf input; route_pts input; num_route_pts input
function Bento_Mission_Dashboard(cur_pos, cur_vel, cur_eul, lidar_x, lidar_y, min_range, num_hits, est_pos, nav_mode, h_agl, vo_conf, mission_phase, active_wp, triage_code, hazard_det, mule_queue, target_pos, sim_time, num_feats, flow_u, flow_v, feat_x, feat_y, s_det, s_pos, s_temp, s_conf, route_pts, num_route_pts)
coder.extrinsic('bentoDashboardLivePlot');
midStart = 37; midEnd = 72;
bentoDashboardLivePlot(cur_pos, cur_vel, cur_eul, lidar_x(midStart:midEnd), lidar_y(midStart:midEnd), min_range, num_hits, est_pos, nav_mode, h_agl, vo_conf, mission_phase, active_wp, triage_code, hazard_det, mule_queue, target_pos, sim_time, num_feats, flow_u, flow_v, feat_x, feat_y, s_det, s_pos, s_temp, s_conf, route_pts, num_route_pts);

== matlab function SAR_Quad_SITL_3D_v3/Visual_Odometry ==
  data: cur_pos input; vo_vel output size=3; cur_vel input; cur_eul input; cur_ang_vel input; sim_time input; vo_conf output size=1; num_feats output size=1; flow_u output size=24; flow_v output size=24; feat_x output size=24; feat_y output size=24
function [vo_vel, vo_conf, num_feats, flow_u, flow_v, feat_x, feat_y] = Visual_Odometry(cur_pos, cur_vel, cur_eul, cur_ang_vel, sim_time)
vo_vel    = zeros(3, 1);
vo_conf   = 0.10;
num_feats = 0.0;
flow_u    = zeros(24, 1);
flow_v    = zeros(24, 1);
feat_x    = zeros(24, 1);
feat_y    = zeros(24, 1);
h_agl     = max(0.0, -cur_pos(3));
persistent p_feat_x p_feat_y feat_init;
if isempty(feat_init)
    feat_init = true; rng(42);
    p_feat_x = 1.4 * (rand(24, 1) - 0.5);
    p_feat_y = 1.4 * (rand(24, 1) - 0.5);
end
feat_x = p_feat_x; feat_y = p_feat_y;
if h_agl >= 0.40
    w_b = [cur_ang_vel(1); cur_ang_vel(2); cur_ang_vel(3)];
    v_b = [cur_vel(1); cur_vel(2); cur_vel(3)];
    R_pitch_cant = [cos(-15*pi/180), 0, sin(-15*pi/180); 0, 1, 0; -sin(-15*pi/180), 0, cos(-15*pi/180)];
    w_c = R_pitch_cant * w_b;
    Z_depth = max(0.8, h_agl);
    v_cam_truth = R_pitch_cant * v_b;
    flow_u = (v_cam_truth(1) - feat_x * v_cam_truth(3)) / Z_depth - (feat_x.*feat_y*w_c(1) - (1 + feat_x.^2)*w_c(2) + feat_y*w_c(3));
    flow_v = (v_cam_truth(2) - feat_y * v_cam_truth(3)) / Z_depth - ((1 + feat_y.^2)*w_c(1) - feat_x.*feat_y*w_c(2) - feat_x*w_c(3));
    derot_u = flow_u + (feat_x.*feat_y.*w_c(1) - (1 + feat_x.^2).*w_c(2) + feat_y*w_c(3));
    derot_v = flow_v + ((1 + feat_y.^2).*w_c(1) - feat_x.*feat_y.*w_c(2) - feat_x*w_c(3));
    calc_vel = R_pitch_cant' * [mean(derot_u) * Z_depth; mean(derot_v) * Z_depth; v_b(3)];
    vo_vel = [calc_vel(1); calc_vel(2); calc_vel(3)];
    vo_conf = 0.90;
    num_feats = 24.0;
end
